simulink model "ClassAandC"  (R2023a)
settings: Solver=VariableStepAuto  StartTime=0.0  StopTime=15  MaxStep=1e-4  RelTol=1e-4  EnableMultiTasking=on
libraries: spsMosfetLib x16, simulink x10, spsDCVoltageSourceLib x9, spsDCMachineLib x5, spsSeriesRLCBranchLib x3, spsDiodeLib x2, spspowerguiLib x1
settings Model: Creator=The MathWorks, Inc.  LastModifiedBy=Admin
settings SolverCC: AlgebraicLoopSolver=TrustRegion
settings DataIOCC: LimitDataPoints=on  SaveFormat=Array  ReturnWorkspaceOutputs=off
settings OptimizationCC: ExpressionDepthLimit=2147483647  InitFltsAndDblsToZero=on  LifeSpan=inf
settings DebuggingCC: SaveWithParameterizedLinksMsg=none  UnderspecifiedInitializationDetection=Classic  MergeDetectMultiDrivingBlocksExec=none  SignalResolutionControl=TryResolveAllWithWarning  SolverPrmCheckMsg=warning  MultiTaskDSMMsg=warning  MultiTaskCondExecSysMsg=none  FcnCallInpInsideContextMsg=warning  UnconnectedInputMsg=warning  UnconnectedOutputMsg=warning  UnconnectedLineMsg=warning  StateNameClashWarn=warning  SFUnexpectedBacktrackingDiag=warning  SFNoUnconditionalDefaultTransitionDiag=warning  SFExecutionAtInitializationDiag=none  ArithmeticOperatorsInVariantConditions=warning
settings HardwareCC: ProdBitPerPointer=32  ProdBitPerSizeT=32  ProdBitPerPtrDiffT=32  ProdLargestAtomicFloat=None  ProdIntDivRoundTo=Undefined  ProdEndianess=Unspecified  ProdWordSize=32  ProdHWDeviceType=32-bit Generic
settings ModelReferenceCC: EnableRefExpFcnMdlSchedulingChecks=on  PropagateSignalLabelsOutOfModel=off
settings SFSimCC: SimUseLocalCustomCode=off  CustomCodeUndefinedFunction=UseInterfaceOnly
settings RTWCC: RTWUseLocalCustomCode=off  DLArmComputeVersion=19.05
settings CodeAppCC: StateflowObjectComments=on
settings GRTTargetCC: TargetFcnLib=ansi_tfl_tmw.mat  TargetLangStandard=C89/C90 (ANSI)  CombineOutputUpdateFcns=off  GRTInterface=on
settings ConfigComp: CovMetricSettings=dw  CovSaveCumulativeToWorkspaceVar=on  CovSaveSingleToWorkspaceVar=on  CovExternalEMLEnable=off  CovSFcnEnable=off
settings SimscapeCC: SimscapeNormalizeSystem=off  SimscapeNominalValues={1, 'bar'; 1, 'cm^3/s'; 1, 'bar*kg/s'; 1, 'kJ/kg'; 1, 'kW'; }

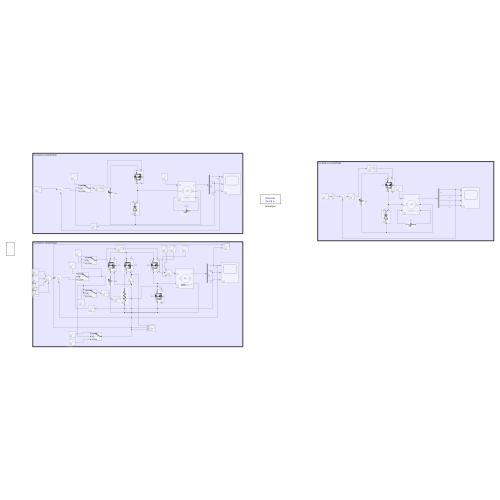
[thumbnail: Simulink's stored preview of the top-level diagram]
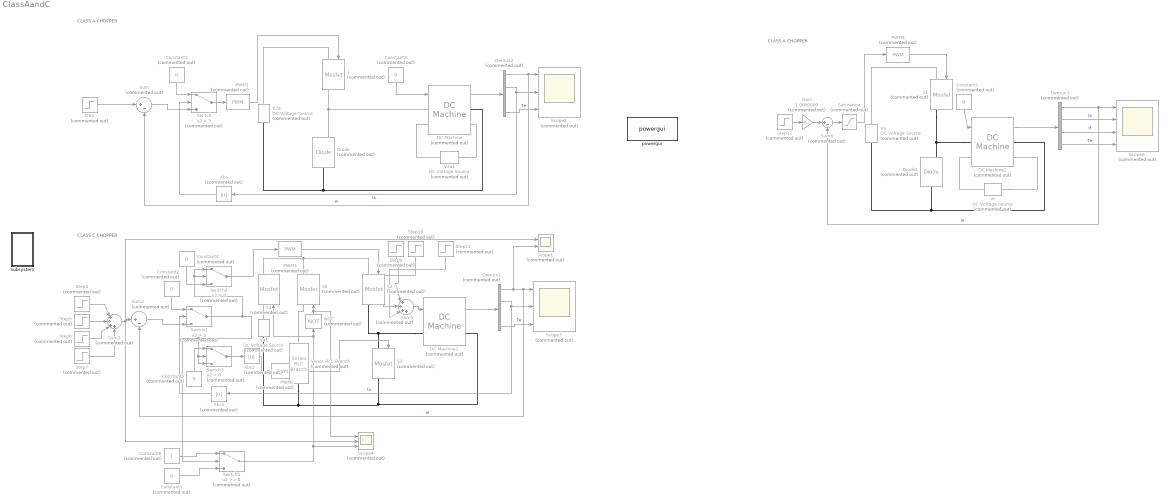
== system ClassAandC ==
  note: CLASS A CHOPPER
  note: CLASS C CHOPPER
  note: CLASS A CHOPPER
  1 : spsMosfetLib/Mosfet  Commented=on  Ron=0.1  Lon=0  Rd=0.01  Vfd=0  IC=0  Rs=1e5  Cs=inf  Measurements=on
  Abs : Abs  Commented=on  SaturateOnIntegerOverflow=off
  Abs1 : Abs  Commented=on  SaturateOnIntegerOverflow=off
  Abs2 : Abs  Commented=on  SaturateOnIntegerOverflow=off
  Constant{1..5,7..8} (7 alike) : Constant  Commented=on  Value=0
  Constant6 : Constant  Commented=on
  DC Machine : spsDCMachineLib/DC Machine  Commented=on  PresetModel=No  MechanicalLoad=Torque TL  FieldType=Wound  ShowDetailedParameters=on  MeasurementBus=off  RLa=[3 0.05]  RLf=[2.02 0.128]  Laf=0.1  MachineConstant=Back-emf constant (V/rpm)  Ke=0.029  Kt=0.27  J=0.012  Bm=0.0006  Tf=0.0958  w0=0  Ifinit=2.47524752475248  TsPowergui=0  TsBlock=-1
  DC Machine1 : spsDCMachineLib/DC Machine  Commented=on  PresetModel=No  MechanicalLoad=Torque TL  FieldType=Permanent magnet  ShowDetailedParameters=on  MeasurementBus=off  RLa=[3 0.05]  RLf=[2.02 0.128]  Laf=0.1  MachineConstant=Back-emf constant (V/rpm)  Ke=0.029  Kt=0.27  J=0.012  Bm=0.0006  Tf=0.0958  w0=0  Ifinit=2.47524752475248  TsPowergui=0  TsBlock=-1
  DC Machine2 : spsDCMachineLib/DC Machine  Commented=on  PresetModel=No  MechanicalLoad=Torque TL  FieldType=Wound  ShowDetailedParameters=on  MeasurementBus=off  RLa=[3 0.05]  RLf=[2.02 0.128]  Laf=0.1  MachineConstant=Back-emf constant (V/rpm)  Ke=0.029  Kt=0.27  J=0.012  Bm=0.0006  Tf=0.0958  w0=0  Ifinit=2.67326732673267  TsPowergui=0  TsBlock=-1
  Demux1 : Demux  Commented=on
  Demux2 : Demux  Commented=on
  Demux3 : Demux  Commented=on
  Diode : spsDiodeLib/Diode  Commented=on  Ron=0.001  Lon=0  Vf=0.8  IC=0  UseSnubber=0  Rs=0  Cs=0  Measurements=on
  Diode1 : spsDiodeLib/Diode  Commented=on  Ron=0.001  Lon=0  Vf=0.8  IC=0  UseSnubber=0  Rs=0  Cs=0  Measurements=on
  Gain : Gain  Commented=on  Gain=1.0000000
  NOT : Logic  Commented=on  Operator=NOT  IconShape=distinctive  AllPortsSameDT=off  OutDataTypeStr=boolean
  PWM{1..4} (4 alike) : simulink/Discontinuities/PWM  Commented=on  DisableCoverage=on  Period=5e-4  InitialDelay=0  DisallowZeroDutyCycle=off  RunAtFixedTimeIntervals=off  SampleTime=0.1
  S{1..5} (5 alike) : spsMosfetLib/Mosfet  Commented=on  Ron=0.1  Lon=0  Rd=0.01  Vfd=0  IC=0  Rs=1e5  Cs=inf  Measurements=on
  Saturation : Saturate  Commented=on  UpperLimit=100  LowerLimit=0
  Scope1 : Scope  Commented=on  NumInputPorts=2
  Scope2 : Scope  Commented=on  NumInputPorts=3
  Scope3 : Scope  Commented=on  NumInputPorts=3
  Scope4 : Scope  Commented=on  NumInputPorts=3
  Scope6 : Scope  Commented=on  NumInputPorts=4
  Series RLC Branch : spsSeriesRLCBranchLib/Series RLC Branch  Commented=on  LConnTagsString=__new0  RConnTagsString=__new0  BranchType=R  Resistance=100000  Inductance=1e-3  SetiL0=off  InitialCurrent=0  Capacitance=1e-6  Setx0=off  InitialVoltage=0  Measurements=None
  Step : Step  Commented=on  After=100  SampleTime=0
  Step10 : Step  Commented=on  Time=5  After=0.1  SampleTime=0
  Step11 : Step  Commented=on  Time=15  After=0.2  SampleTime=0
  Step12 : Step  Commented=on  After=100  SampleTime=0
  Step4 : Step  Commented=on  After=100  SampleTime=0
  Step5 : Step  Commented=on  Time=8  After=200  SampleTime=0
  Step6 : Step  Commented=on  Time=15  After=-150  SampleTime=0
  Step7 : Step  Commented=on  Time=25  After=-150  SampleTime=0
  Step9 : Step  Commented=on  Time=3  After=0.3  SampleTime=0
  Subsystem : Subsystem
  Sum : Sum  Commented=on  Inputs=|+-
  Sum2 : Sum  Commented=on  Inputs=|+-
  Sum3 : Sum  Commented=on  Inputs=|++++
  Sum5 : Sum  Commented=on  Inputs=|++++
  Sum6 : Sum  Commented=on  Inputs=|+-
  Switch : Switch  Commented=on  Criteria=u2 > Threshold  Threshold=3  SaturateOnIntegerOverflow=off  InputSameDT=off
  Switch1 : Switch  Commented=on  Criteria=u2 > Threshold  Threshold=3  SaturateOnIntegerOverflow=off  InputSameDT=off
  Switch2 : Switch  Commented=on  Criteria=u2 > Threshold  SaturateOnIntegerOverflow=off  InputSameDT=off
  Switch3 : Switch  Commented=on  Criteria=u2 > Threshold  SaturateOnIntegerOverflow=off  InputSameDT=off
  Switch4 : Switch  Commented=on  SaturateOnIntegerOverflow=off  InputSameDT=off
  V2a : spsDCVoltageSourceLib/DC Voltage Source  Commented=on  Amplitude=200  Measurements=None
  V2a1 : spsDCVoltageSourceLib/DC Voltage Source  Commented=on  Amplitude=200  Measurements=None
  Va : spsDCVoltageSourceLib/DC Voltage Source  Commented=on  Amplitude=85  Measurements=None
  Va1 : spsDCVoltageSourceLib/DC Voltage Source  Commented=on  Amplitude=200  Measurements=None
  Vt : spsDCVoltageSourceLib/DC Voltage Source  Commented=on  Amplitude=5.4  Measurements=None
  powergui : spspowerguiLib/powergui  SimulationMode=Discrete  SampleTime=20e-6  frequency=60  Iterations=50  frequencyindice=0  Pbase=100e6  ErrMax=1e-4  UnitsV=kV  UnitsW=MW  buscounter=0  FunctionMessages=off  echomessages=off  EnableUseOfTLC=off  CurrentSourceSwitches=off  DisableSnubberDevices=off  DisableRonSwitches=off  DisableVfSwitches=off  DisplayEquations=off  AutomaticDiscreteSolvers=off  SolverType=Tustin/Backward Euler (TBE)  Interpol=off  ExternalGateDelay=off  methode=off  Ts=100  x0status=blocks  SPID=on  SwTol=0  HookPort=off  NonlinearTolerance=1e-4  nMaxIteration=100  ContinueOnMaxIteration=off  RestoreLinks=warning  ResistiveCurrentMeasurement=off  Frange=[0:2:500]  Ylog=off  Xlog=on  ShowGrid=off  save=off  variable=ZData  structure=0  ZoomFFT=on  StartTime=0.0  cycles=1  DisplayStyle=1  fundamental=60  FreqAxis=off  MaxFrequency=1000  frequencyindicesteady=1  RmsSteady=1  display=off
  wires:
  Demux2/4 -> Scope2/3  "Te"
  Demux2/2 -> Scope2/2, Abs/1  "Ia"
  Demux2/1 -> Scope2/1, Sum/2  "w"
  DC Machine/1 -> Demux2/1
  PWM1/1 -> 1/1
  Constant3/1 -> Switch/1
  Switch/1 -> PWM1/1
  Sum/1 -> Switch/3
  Abs/1 -> Switch/2
  Step/1 -> Sum/1
  Step5/1 -> Sum3/2
  Sum3/1 -> Scope1/1, Scope4/2, Sum2/1
  Sum2/1 -> Switch1/3
  Step6/1 -> Sum3/3
  Step7/1 -> Sum3/4
  Constant2/1 -> Switch1/1
  Abs1/1 -> Switch1/2
  Demux1/4 -> Scope3/3  "Te"
  Demux1/1 -> Scope1/2, Scope3/1, Sum2/2  "w"
  Step4/1 -> Sum3/1
  DC Machine1/1 -> Demux1/1
  Demux1/2 -> Scope3/2, Abs1/1  "Ia"
  Switch1/1 -> Switch4/2, Switch3/3, Switch3/2, Switch2/1, Switch2/2
  Constant4/1 -> Switch2/3
  Switch2/1 -> PWM3/1
  Constant5/1 -> Switch3/1
  Switch3/1 -> Abs2/1
  PWM3/1 -> S2/1
  Abs2/1 -> PWM2/1
  PWM2/1 -> S3/1
  NOT/1 -> Scope4/1, S5/1
  Constant6/1 -> Switch4/1
  Constant7/1 -> Switch4/3
  Switch4/1 -> S4/1, NOT/1, Scope4/3
  Step9/1 -> Sum5/1
  Sum5/1 -> DC Machine1/1
  Step11/1 -> Sum5/3
  Step10/1 -> Sum5/2
  Demux3/2 -> Scope6/2  "Ia"
  DC Machine2/1 -> Demux3/1
  Demux3/4 -> Scope6/4  "Te"
  Demux3/3 -> Scope6/3  "If"
  PWM4/1 -> S1/1
  Demux3/1 -> Sum6/2, Scope6/1  "w"
  Constant1/1 -> DC Machine2/1
  Sum6/1 -> Saturation/1
  Saturation/1 -> PWM4/1
  Step12/1 -> Gain/1
  Gain/1 -> Sum6/1
  Constant8/1 -> DC Machine/1
  connections:
  1/RConn1 -- Diode/RConn1 -- DC Machine/LConn1
  Diode/LConn1 -- V2a/LConn1 -- DC Machine/RConn1
  1/LConn1 -- V2a/RConn1
  DC Machine1/LConn1 -- S2/RConn1 -- S3/LConn1
  DC Machine1/RConn1 -- Series RLC Branch/RConn1 -- Va1/LConn1 -- S3/RConn1
  S4/LConn1 -- Va1/RConn1
  S4/RConn1 -- S5/RConn1 -- S2/LConn1
  Series RLC Branch/LConn1 -- S5/LConn1
  DC Machine2/LConn1 -- S1/RConn1 -- Diode1/RConn1
  DC Machine2/RConn1 -- Va/LConn1 -- Diode1/LConn1
  S1/LConn1 -- Va/RConn1
  Vt/RConn1 -- DC Machine2/LConn2
  Vt/LConn1 -- DC Machine2/RConn2
  V2a1/LConn1 -- DC Machine/RConn2
  V2a1/RConn1 -- DC Machine/LConn2

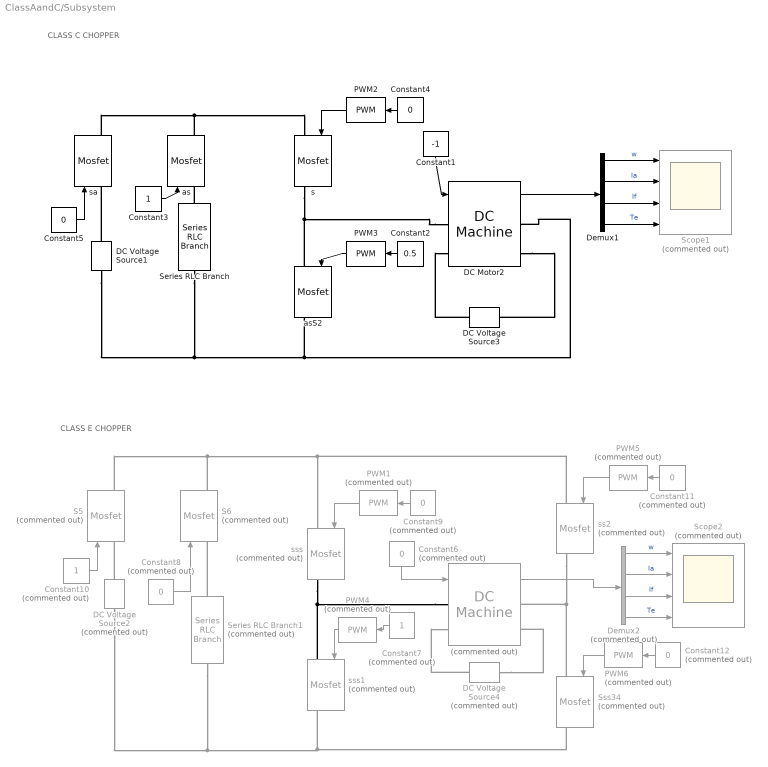
== system ClassAandC/Subsystem ==
  note: CLASS C CHOPPER
  note: CLASS E CHOPPER
  " " : spsDCMachineLib/DC Machine  Commented=on  PresetModel=No  MechanicalLoad=Torque TL  FieldType=Wound  ShowDetailedParameters=on  MeasurementBus=off  RLa=[3 0.05]  RLf=[2.02 0.128]  Laf=0.1  MachineConstant=Back-emf constant (V/rpm)  Ke=0.029  Kt=0.27  J=0.012  Bm=0.0006  Tf=0.0958  w0=0  Ifinit=2.67326732673267  TsPowergui=0  TsBlock=-1
  Constant1 : Constant  Value=-1
  Constant10 : Constant  Commented=on
  Constant{6,8..9,11..12} (5 alike) : Constant  Commented=on  Value=0
  Constant2 : Constant  Value=0.5
  Constant3 : Constant
  Constant4 : Constant  Value=0
  Constant5 : Constant  Value=0
  Constant7 : Constant  Commented=on
  DC Motor2 : spsDCMachineLib/DC Machine  PresetModel=No  MechanicalLoad=Torque TL  FieldType=Wound  ShowDetailedParameters=on  MeasurementBus=off  RLa=[3.1 0.05]  RLf=[2.02 0.128]  Laf=0.1  MachineConstant=Back-emf constant (V/rpm)  Ke=0.029  Kt=0.27  J=0.012  Bm=0.0006  Tf=0.0958  w0=0  Ifinit=2.67326732673267  TsPowergui=0  TsBlock=-1
  DC Voltage Source1 : spsDCVoltageSourceLib/DC Voltage Source  Amplitude=85  Measurements=None
  DC Voltage Source2 : spsDCVoltageSourceLib/DC Voltage Source  Commented=on  Amplitude=85  Measurements=None
  DC Voltage Source3 : spsDCVoltageSourceLib/DC Voltage Source  Amplitude=5.4  Measurements=None
  DC Voltage Source4 : spsDCVoltageSourceLib/DC Voltage Source  Commented=on  Amplitude=5.4  Measurements=None
  Demux1 : Demux
  Demux2 : Demux  Commented=on
  PWM{1,4..6} (4 alike) : simulink/Discontinuities/PWM  Commented=on  DisableCoverage=on  Period=5e-4  InitialDelay=0  DisallowZeroDutyCycle=off  RunAtFixedTimeIntervals=off  SampleTime=0.1
  PWM2 : simulink/Discontinuities/PWM  DisableCoverage=on  Period=5e-4  InitialDelay=0  DisallowZeroDutyCycle=off  RunAtFixedTimeIntervals=off  SampleTime=0.1
  PWM3 : simulink/Discontinuities/PWM  DisableCoverage=on  Period=5e-4  InitialDelay=0  DisallowZeroDutyCycle=off  RunAtFixedTimeIntervals=off  SampleTime=0.1
  S5 : spsMosfetLib/Mosfet  Commented=on  Ron=0.1  Lon=0  Rd=0.01  Vfd=0  IC=0  Rs=1e5  Cs=inf  Measurements=on
  S6 : spsMosfetLib/Mosfet  Commented=on  Ron=0.1  Lon=0  Rd=0.01  Vfd=0  IC=0  Rs=1e5  Cs=inf  Measurements=on
  Scope1 : Scope  Commented=on  NumInputPorts=4
  Scope2 : Scope  Commented=on  NumInputPorts=4
  Series RLC Branch : spsSeriesRLCBranchLib/Series RLC Branch  LConnTagsString=__new0  RConnTagsString=__new0  BranchType=R  Resistance=20  Inductance=1e-3  SetiL0=off  InitialCurrent=0  Capacitance=1e-6  Setx0=off  InitialVoltage=0  Measurements=None
  Series RLC Branch1 : spsSeriesRLCBranchLib/Series RLC Branch  Commented=on  LConnTagsString=__new0  RConnTagsString=__new0  BranchType=R  Resistance=20  Inductance=1e-3  SetiL0=off  InitialCurrent=0  Capacitance=1e-6  Setx0=off  InitialVoltage=0  Measurements=None
  Sss34 : spsMosfetLib/Mosfet  Commented=on  Ron=0.1  Lon=0  Rd=0.01  Vfd=0  IC=0  Rs=1e5  Cs=inf  Measurements=on
  as : spsMosfetLib/Mosfet  Ron=0.1  Lon=0  Rd=0.01  Vfd=0  IC=0  Rs=1e5  Cs=inf  Measurements=on
  asS2 : spsMosfetLib/Mosfet  Ron=0.1  Lon=0  Rd=0.01  Vfd=0  IC=0  Rs=1e5  Cs=inf  Measurements=on
  s : spsMosfetLib/Mosfet  Ron=0.1  Lon=0  Rd=0.01  Vfd=0  IC=0  Rs=1e5  Cs=inf  Measurements=on
  sa : spsMosfetLib/Mosfet  Ron=0.1  Lon=0  Rd=0.01  Vfd=0  IC=0  Rs=1e5  Cs=inf  Measurements=on
  ss2 : spsMosfetLib/Mosfet  Commented=on  Ron=0.1  Lon=0  Rd=0.01  Vfd=0  IC=0  Rs=1e5  Cs=inf  Measurements=on
  sss : spsMosfetLib/Mosfet  Commented=on  Ron=0.1  Lon=0  Rd=0.01  Vfd=0  IC=0  Rs=1e5  Cs=inf  Measurements=on
  sss1 : spsMosfetLib/Mosfet  Commented=on  Ron=0.1  Lon=0  Rd=0.01  Vfd=0  IC=0  Rs=1e5  Cs=inf  Measurements=on
  wires:
  DC Motor2/1 -> Demux1/1
  PWM2/1 -> s/1
  PWM3/1 -> asS2/1
  Constant1/1 -> DC Motor2/1
  Demux1/3 -> Scope1/3  "If"
  Demux1/2 -> Scope1/2  "Ia"
  Demux1/4 -> Scope1/4  "Te"
  Constant2/1 -> PWM3/1
  Demux1/1 -> Scope1/1  "w"
  Constant4/1 -> PWM2/1
  Constant3/1 -> as/1
  Constant5/1 -> sa/1
  Constant10/1 -> S5/1
  Constant8/1 -> S6/1
  Constant9/1 -> PWM1/1
  Demux2/1 -> Scope2/1  "w"
  Constant7/1 -> PWM4/1
  Demux2/4 -> Scope2/4  "Te"
  Demux2/2 -> Scope2/2  "Ia"
  Demux2/3 -> Scope2/3  "If"
  Constant6/1 -> " "/1
  PWM4/1 -> sss1/1
  PWM1/1 -> sss/1
  " "/1 -> Demux2/1
  PWM5/1 -> ss2/1
  Constant11/1 -> PWM5/1
  Constant12/1 -> PWM6/1
  PWM6/1 -> Sss34/1
  connections:
  DC Motor2/LConn1 -- asS2/LConn1 -- s/RConn1
  asS2/RConn1 -- Series RLC Branch/RConn1 -- DC Voltage Source1/LConn1 -- DC Motor2/RConn1
  sa/RConn1 -- as/RConn1 -- s/LConn1
  DC Voltage Source1/RConn1 -- sa/LConn1
  Series RLC Branch/LConn1 -- as/LConn1
  " "/LConn1 -- sss1/LConn1 -- sss/RConn1
  Series RLC Branch1/RConn1 -- DC Voltage Source2/LConn1 -- Sss34/RConn1 -- sss1/RConn1
  S5/RConn1 -- S6/RConn1 -- ss2/LConn1 -- sss/LConn1
  DC Voltage Source2/RConn1 -- S5/LConn1
  Series RLC Branch1/LConn1 -- S6/LConn1
  ss2/RConn1 -- Sss34/LConn1 -- " "/RConn1
  DC Voltage Source3/RConn1 -- DC Motor2/LConn2
  DC Voltage Source4/RConn1 -- " "/LConn2
  DC Voltage Source4/LConn1 -- " "/RConn2
  DC Motor2/RConn2 -- DC Voltage Source3/LConn1
